simulink model "example7_10"  (R2016b)
settings: Solver=ode45  StartTime=0.0  StopTime=15  RelTol=1e-3
libraries: commdigbbndfm2 x2, commchan3 x1, commrandsrc3 x1, commsink2 x1
settings Model: Creator=zhangjin  LastModifiedBy=zhangjin

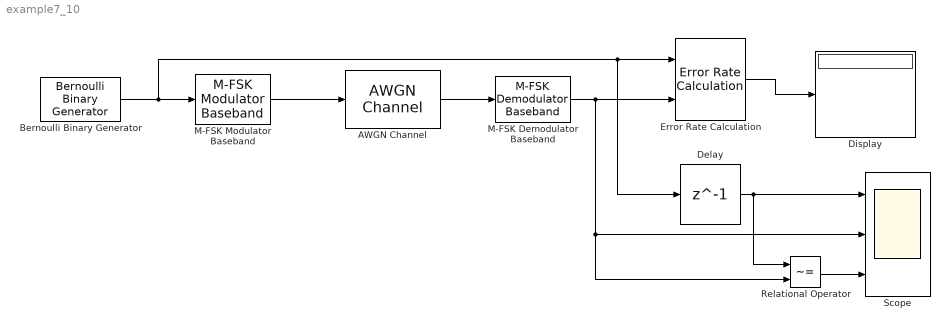
== system example7_10 ==
  AWGN Channel : commchan3/AWGN Channel  InputProcessing=Inherited (this choice will be removed - see release notes)  seed=113  noiseMode="Signal to noise ratio  (Eb/No)"  EbNodB=10  EsNodB=10  SNRdB=10  bitsPerSym=1  Ps=1  Tsym=1/1200  variance=1
  Bernoulli Binary Generator : commrandsrc3/Bernoulli Binary Generator  ProbabilityOfZero=0.5  SeedSource=Parameter  Seed=89  SampleTime=1/1200  SamplesPerFrame=1  OutputDataType=double  SimulateUsing=Interpreted execution
  Delay : Delay  DelayLength=1  InputProcessing=Columns as channels (frame based)
  Display : Display
  Error Rate Calculation : commsink2/Error Rate Calculation  N=1  st_delay=0  cp_mode=Entire frame  subframe=[]  PMode=Port  WsName=ErrorVec  RsMode2=off  stop=off  numErr=100  maxBits=1e6
  M-FSK Demodulator Baseband : commdigbbndfm2/M-FSK Demodulator Baseband  M=2  OutType=Integer  Dec=Binary  freqSep=1000  numSamp=5  RateOptions=Inherit from input (this choice will be removed - see release notes)  outDataType=double
  M-FSK Modulator Baseband : commdigbbndfm2/M-FSK Modulator Baseband  M=2  InType=Integer  Enc=Binary  freqSep=1000  phaseType=Continuous  numSamp=5  RateOptions=Inherit from input (this choice will be removed - see release notes)  outDataType=single
  Relational Operator : RelationalOperator  Operator=~=  OutDataTypeStr=boolean  RndMeth=Simplest
  Scope : Scope  NumInputPorts=3
  wires:
  Bernoulli Binary Generator/1 -> Delay/1, Error Rate Calculation/1, M-FSK Modulator Baseband/1
  M-FSK Modulator Baseband/1 -> AWGN Channel/1
  AWGN Channel/1 -> M-FSK Demodulator Baseband/1
  M-FSK Demodulator Baseband/1 -> Relational Operator/2, Scope/2, Error Rate Calculation/2
  Error Rate Calculation/1 -> Display/1
  Delay/1 -> Relational Operator/1, Scope/1
  Relational Operator/1 -> Scope/3
